simulink model "myFirstController_sim"  (R2014a)
settings: Solver=ode45  StartTime=0.0  StopTime=15  RelTol=1e-3
values from neighbouring files (symbols this model uses):
  A = [0.7115  -0.4345; 0.4345  0.8853]    [myFirstController_data.mat]
  B = [0.2173 0.0573]    [myFirstController_data.mat]
  C_all = [1  0; 0  1]    [myFirstController_data.mat]
settings Model: Creator=Juan  LastModifiedBy=juanj
settings DataIOCC: SignalLoggingSaveFormat=ModelDataLogs
settings DebuggingCC: UnderspecifiedInitializationDetection=Classic  MultiTaskDSMMsg=warning  MultiTaskCondExecSysMsg=none  StateNameClashWarn=warning  StrictBusMsg=None
settings RTWCC: IncludeERTFirstTime=on

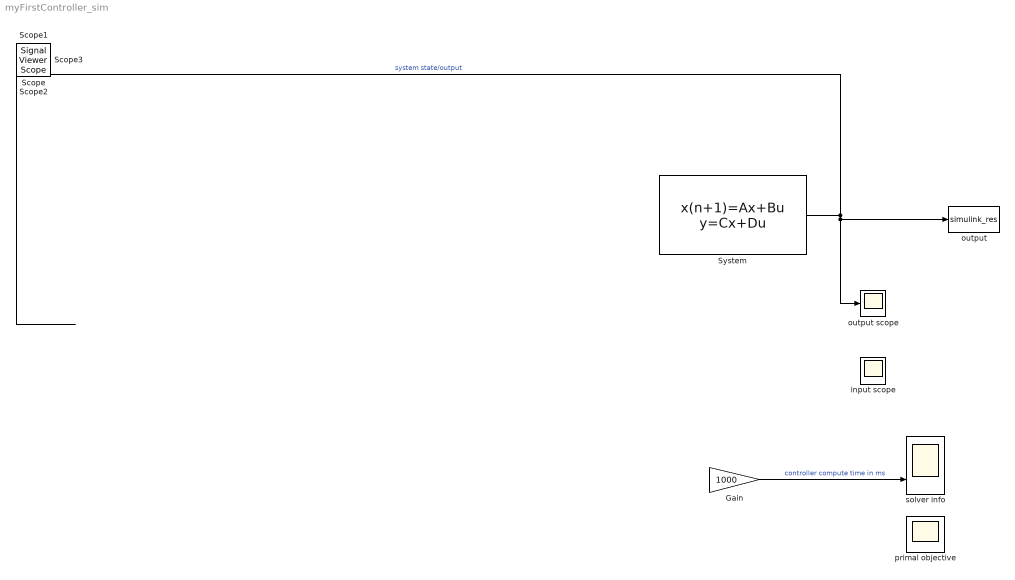
== system myFirstController_sim ==
  Gain : Gain  Gain=1000
  System : DiscreteStateSpace  A=A  B=B  C=C_all  D=zeros(2,1)  X0=[0; 6]
  input scope : Scope
      settings: TimeRange=140  YMin=-26  YMax=26  SaveName=ScopeData4
  output : ToWorkspace  VariableName=simulink_res  SaveFormat=Timeseries  SampleTime=-1
  output scope : Scope
      settings: TimeRange=140  YMin=-26  YMax=26
  primal objective : Scope
      settings: TimeRange=140  YMin=-26  YMax=26  SaveName=ScopeData3
  solver info : Scope  NumInputPorts=2
      settings: TimeRange=140  YMin=22~0.9  YMax=26~1.6  SaveName=ScopeData2
  Scope : SignalViewerScope  IOType=viewer  ZoomMode=yonly  RefreshTime=0.035000
      settings: YMin=-25  YMax=25
  Scope1 : SignalViewerScope  IOType=viewer  RefreshTime=0.035000
  Scope2 : SignalViewerScope  IOType=viewer  RefreshTime=0.035000
      settings: SaveName=ScopeData2
  Scope3 : SignalViewerScope  IOType=viewer  RefreshTime=0.035000
      settings: SaveName=ScopeData3
  wires:
  System/1 -> output scope/1, output/1  "system state/output"
  ? -> System/1, input scope/1  "optimal input"
  ? -> Gain/1
  Gain/1 -> solver info/2  "controller compute time in ms"
  ? -> solver info/1  "number of iterations"
  ? -> primal objective/1  "primal objective"
